simulink model "LL_rdf1"  (R2013b)
settings: Solver=ode45  StartTime=0.0  StopTime=40.0  MaxStep=0.5  RelTol=1e-3
settings Model: Creator=rmg37  LastModifiedBy=rmg37

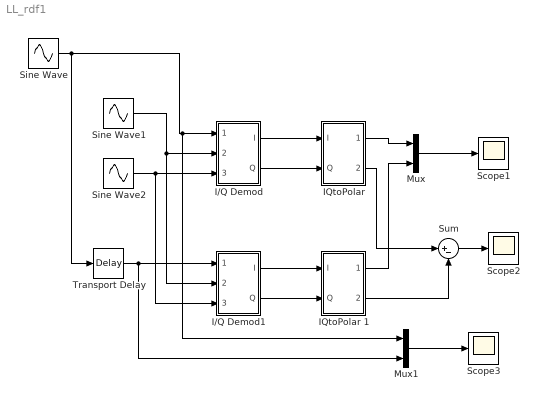
== system LL_rdf1 ==
  I/Q Demod : Subsystem
  I/Q Demod1 : Subsystem
  "IQtoPolar " : Subsystem
  IQtoPolar 1 : Subsystem
  Mux : Mux  Inputs=2
  Mux1 : Mux  Inputs=2
  Scope1 : Scope
  Scope2 : Scope
  Scope3 : Scope
      settings: SaveName=ScopeData2
  Sine Wave : Sin  Frequency=2*pi*99.9  SampleTime=0
  Sine Wave1 : Sin  Frequency=2*pi*100  SampleTime=0
  Sine Wave2 : Sin  Frequency=2*pi*100  Phase=pi/2  SampleTime=0
  Sum : Sum  Inputs=|+-
  Transport Delay : TransportDelay  DelayTime=1/600
  wires:
  I/Q Demod/1(I) -> "IQtoPolar "/1(I)
  I/Q Demod/2(Q) -> "IQtoPolar "/2(Q)
  Sine Wave/1 -> Transport Delay/1, Mux1/1, I/Q Demod/1(RF in)
  Sine Wave1/1 -> I/Q Demod1/2(LO_I), I/Q Demod/2(LO_I)
  Sine Wave2/1 -> I/Q Demod1/3("LO_Q "), I/Q Demod/3("LO_Q ")
  "IQtoPolar "/1(Mag) -> Mux/1
  Mux/1 -> Scope1/1
  I/Q Demod1/1(I) -> IQtoPolar 1/1(I)
  I/Q Demod1/2(Q) -> IQtoPolar 1/2(Q)
  Transport Delay/1 -> Mux1/2, I/Q Demod1/1(RF in)
  IQtoPolar 1/1(Mag) -> Mux/2
  "IQtoPolar "/2(Phase) -> Sum/1
  IQtoPolar 1/2(Phase) -> Sum/2
  Sum/1 -> Scope2/1
  Mux1/1 -> Scope3/1

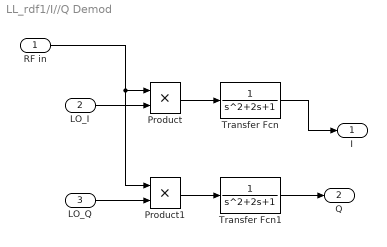
== system LL_rdf1/I//Q Demod ==
  RF in : Inport
  LO_I : Inport  Port=2
  "LO_Q " : Inport  Port=3
  Product : Product
  Product1 : Product
  Transfer Fcn : TransferFcn
  Transfer Fcn1 : TransferFcn
  I : Outport
  Q : Outport  Port=2
  wires:
  LO_I/1 -> Product/2
  Product/1 -> Transfer Fcn/1
  Transfer Fcn/1 -> I/1
  "LO_Q "/1 -> Product1/2
  Product1/1 -> Transfer Fcn1/1
  Transfer Fcn1/1 -> Q/1
  RF in/1 -> Product1/1, Product/1

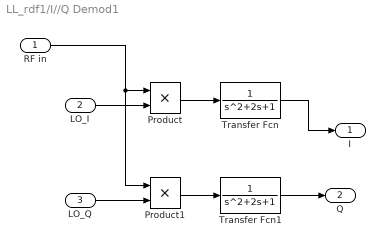
== system LL_rdf1/I//Q Demod1 ==
  RF in : Inport
  LO_I : Inport  Port=2
  "LO_Q " : Inport  Port=3
  Product : Product
  Product1 : Product
  Transfer Fcn : TransferFcn
  Transfer Fcn1 : TransferFcn
  I : Outport
  Q : Outport  Port=2
  wires:
  LO_I/1 -> Product/2
  Product/1 -> Transfer Fcn/1
  Transfer Fcn/1 -> I/1
  "LO_Q "/1 -> Product1/2
  Product1/1 -> Transfer Fcn1/1
  Transfer Fcn1/1 -> Q/1
  RF in/1 -> Product1/1, Product/1

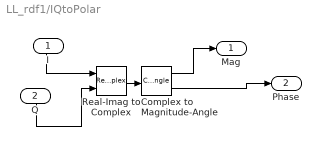
== system LL_rdf1/IQtoPolar  ==
  I : Inport
  Q : Inport  Port=2
  Complex to Magnitude-Angle : ComplexToMagnitudeAngle
  Real-Imag to Complex : RealImagToComplex
  Mag : Outport
  Phase : Outport  Port=2
  wires:
  Q/1 -> Real-Imag to Complex/2
  I/1 -> Real-Imag to Complex/1
  Complex to Magnitude-Angle/1 -> Mag/1
  Complex to Magnitude-Angle/2 -> Phase/1
  Real-Imag to Complex/1 -> Complex to Magnitude-Angle/1

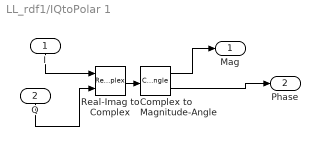
== system LL_rdf1/IQtoPolar 1 ==
  I : Inport
  Q : Inport  Port=2
  Complex to Magnitude-Angle : ComplexToMagnitudeAngle
  Real-Imag to Complex : RealImagToComplex
  Mag : Outport
  Phase : Outport  Port=2
  wires:
  Q/1 -> Real-Imag to Complex/2
  I/1 -> Real-Imag to Complex/1
  Complex to Magnitude-Angle/1 -> Mag/1
  Complex to Magnitude-Angle/2 -> Phase/1
  Real-Imag to Complex/1 -> Complex to Magnitude-Angle/1
